simulink model "Q6_b"  (R2017a)
settings: Solver=FixedStepAuto  StartTime=0.0  StopTime=10  FixedStep=0.01  RelTol=0.00001
model workspace (MAT data in the model file):
  Kp_1 = 10000
  Kp_2 = 10000
  Kv_1 = 200
  Kv_2 = 200
  a_1 = 1
  a_2 = 1
  g = 9.8
  m_1 = 1
  m_2 = 1
  q1_0 = 0
  q1_dot_0 = 0
  q1_dot_f = 0
  q1_double_dot_0 = 0
  q1_double_dot_f = 0
  q1_f = 0.523598775598
  q2_0 = 0
  q2_dot_0 = 0
  q2_dot_f = 0
  q2_double_dot_0 = 0
  q2_double_dot_f = 0
  q2_f = 2.09439510239
  simulation_time = 4
libraries: simulink x25
settings Model: Creator=Omer  LastModifiedBy=Omer
settings ModelReferenceCC: ModelReferenceMinAlgLoopOccurrences=on

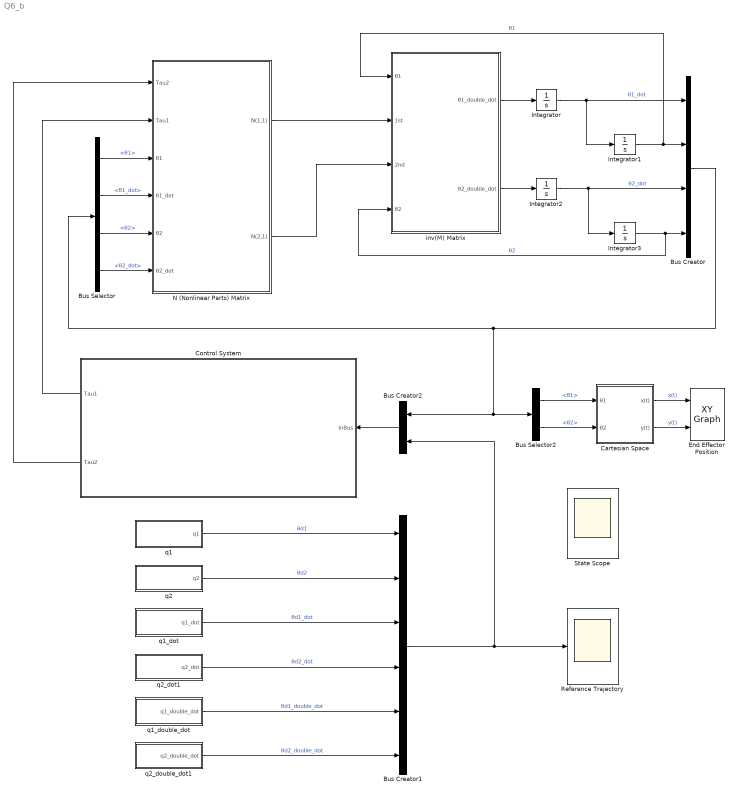
== system Q6_b ==
  Bus Creator : BusCreator  Inputs=4
  Bus Creator1 : BusCreator  Inputs=6
  Bus Creator2 : BusCreator  Inputs=2
  Bus Selector : BusSelector  OutputSignals=θ1,θ1_dot,θ2,θ2_dot
  Bus Selector2 : BusSelector  OutputSignals=θ1,θ2
  "Cartesian Space " : Subsystem  TreatAsAtomicUnit=on
  Control System : Subsystem  TreatAsAtomicUnit=on
  End Effector Position : simulink/Sinks/XY Graph  xmin=-1  xmax=3  ymin=-1  ymax=2  st=-1
  Integrator{,1..3} (4 alike) : Integrator
  N (Nonlinear Parts) Matrix : Subsystem  TreatAsAtomicUnit=on
  Reference Trajectory : Scope
  State Scope : Scope
      settings: Floating=on
  inv(M) Matrix : Subsystem  TreatAsAtomicUnit=on
  q1 : Subsystem  TreatAsAtomicUnit=on
  q1_dot : Subsystem  TreatAsAtomicUnit=on
  q1_double_dot : Subsystem  TreatAsAtomicUnit=on
  q2 : Subsystem  TreatAsAtomicUnit=on
  q2_dot1 : Subsystem  TreatAsAtomicUnit=on
  q2_double_dot1 : Subsystem  TreatAsAtomicUnit=on
  wires:
  N (Nonlinear Parts) Matrix/2(N(2,1)) -> inv(M) Matrix/3(2nd)
  N (Nonlinear Parts) Matrix/1(N(1,1)) -> inv(M) Matrix/2(1st)
  Bus Creator/1 -> Bus Selector/1, Bus Creator2/1, Bus Selector2/1
  inv(M) Matrix/2(θ2_double_dot) -> Integrator2/1
  Bus Selector/1 -> N (Nonlinear Parts) Matrix/3("θ1 ")  "<θ1>"
  Integrator2/1 -> Integrator3/1, Bus Creator/3  "θ2_dot"
  Integrator3/1 -> inv(M) Matrix/4(θ2), Bus Creator/4  "θ2"
  Integrator1/1 -> inv(M) Matrix/1(θ1), Bus Creator/2  "θ1"
  Bus Selector/3 -> N (Nonlinear Parts) Matrix/5(θ2)  "<θ2>"
  Bus Selector/2 -> N (Nonlinear Parts) Matrix/4(θ1_dot)  "<θ1_dot>"
  Integrator/1 -> Bus Creator/1, Integrator1/1  "θ1_dot"
  Bus Selector/4 -> N (Nonlinear Parts) Matrix/6(θ2_dot)  "<θ2_dot>"
  inv(M) Matrix/1(θ1_double_dot) -> Integrator/1
  Bus Selector2/1 -> "Cartesian Space "/1(θ1)  "<θ1>"
  Bus Selector2/2 -> "Cartesian Space "/2(θ2)  "<θ2>"
  "Cartesian Space "/1(x(t)) -> End Effector Position/1  "x(t)"
  "Cartesian Space "/2(y(t)) -> End Effector Position/2  "y(t)"
  Bus Creator2/1 -> Control System/1(InBus)
  Bus Creator1/1 -> Bus Creator2/2, Reference Trajectory/1
  q1/1(q1) -> Bus Creator1/1  "θd1"
  q2/1(q2) -> Bus Creator1/2  "θd2"
  Control System/2(Tau2) -> N (Nonlinear Parts) Matrix/1(Tau2)
  Control System/1(Tau1) -> N (Nonlinear Parts) Matrix/2(Tau1)
  q1_dot/1(q1_dot) -> Bus Creator1/3  "θd1_dot"
  q2_dot1/1(q2_dot) -> Bus Creator1/4  "θd2_dot"
  q1_double_dot/1(q1_double_dot) -> Bus Creator1/5  "θd1_double_dot"
  q2_double_dot1/1(q2_double_dot) -> Bus Creator1/6  "θd2_double_dot"

== system Q6_b/Cartesian Space  ==
  θ1 : Inport
  θ2 : Inport  Port=2
  Gain : Gain  Gain=a_1
  Gain1 : Gain  Gain=a_1
  Gain2 : Gain  Gain=a_2
  Gain3 : Gain  Gain=a_2
  Sum : Sum  Inputs=++|
  Sum1 : Sum  Inputs=|++
  Sum2 : Sum  Inputs=+|+
  Trig Func : Trigonometry
  Trig Func1 : Trigonometry
  Trig Func2 : Trigonometry  Operator=cos
  Trig Func3 : Trigonometry  Operator=cos
  x(t) : Outport
  y(t) : Outport  Port=2
  wires:
  θ1/1 -> Trig Func2/1, Trig Func/1, Sum/1
  θ2/1 -> Sum/2
  Sum/1 -> Trig Func3/1, Trig Func1/1
  Sum2/1 -> y(t)/1
  Sum1/1 -> x(t)/1
  Trig Func/1 -> Gain/1
  Gain/1 -> Sum2/1
  Trig Func2/1 -> Gain1/1
  Gain1/1 -> Sum1/1
  Trig Func1/1 -> Gain2/1
  Gain2/1 -> Sum2/2
  Trig Func3/1 -> Gain3/1
  Gain3/1 -> Sum1/2

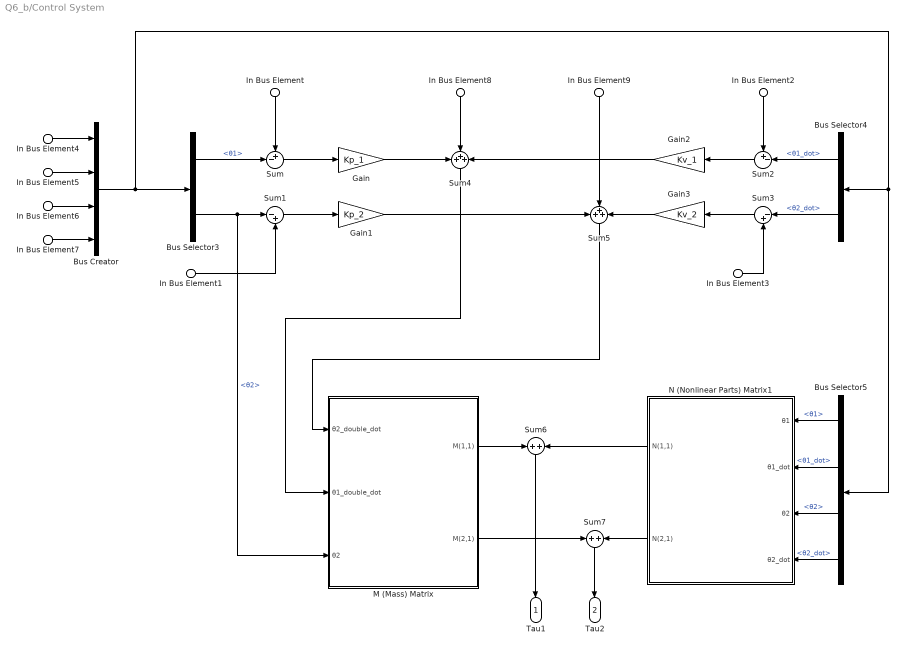
== system Q6_b/Control System ==
  In Bus Element : Inport  PortName=InBus  Element=signal2.θd1
  In Bus Element1 : Inport  PortName=InBus  Element=signal2.θd2
  In Bus Element2 : Inport  PortName=InBus  Element=signal2.θd1_dot
  In Bus Element3 : Inport  PortName=InBus  Element=signal2.θd2_dot
  In Bus Element8 : Inport  PortName=InBus  Element=signal2.θd1_double_dot
  In Bus Element9 : Inport  PortName=InBus  Element=signal2.θd2_double_dot
  In Bus Element4 : Inport  PortName=InBus  Element=signal1.θ1_dot
  In Bus Element5 : Inport  PortName=InBus  Element=signal1.θ1
  In Bus Element6 : Inport  PortName=InBus  Element=signal1.θ2_dot
  In Bus Element7 : Inport  PortName=InBus  Element=signal1.θ2
  Bus Creator : BusCreator  Inputs=4
  Bus Selector3 : BusSelector  OutputSignals=θ1,θ2
  Bus Selector4 : BusSelector  OutputSignals=θ1_dot,θ2_dot
  Bus Selector5 : BusSelector  OutputSignals=θ1,θ1_dot,θ2,θ2_dot
  Gain : Gain  Gain=Kp_1
  Gain1 : Gain  Gain=Kp_2
  Gain2 : Gain  Gain=Kv_1
  Gain3 : Gain  Gain=Kv_2
  M (Mass) Matrix : Subsystem  TreatAsAtomicUnit=on
  N (Nonlinear Parts) Matrix1 : Subsystem  TreatAsAtomicUnit=on
  Sum : Sum  Inputs=+-|
  Sum1 : Sum  Inputs=|-+
  Sum2 : Sum  Inputs=+-|
  Sum3 : Sum  Inputs=|-+
  Sum4 : Sum  Inputs=+++
  Sum5 : Sum  Inputs=+++
  Sum6 : Sum  Inputs=+|+
  Sum7 : Sum  Inputs=+|+
  Tau1 : Outport
  Tau2 : Outport  Port=2
  wires:
  Sum4/1 -> M (Mass) Matrix/2(θ1_double_dot)
  M (Mass) Matrix/1(M(1,1)) -> Sum6/1
  In Bus Element1/1 -> Sum1/2
  Sum7/1 -> Tau2/1
  In Bus Element7/1 -> Bus Creator/4
  In Bus Element3/1 -> Sum3/2
  N (Nonlinear Parts) Matrix1/1(N(1,1)) -> Sum6/2
  In Bus Element5/1 -> Bus Creator/2
  Gain1/1 -> Sum5/1
  In Bus Element4/1 -> Bus Creator/1
  Sum3/1 -> Gain3/1
  Sum2/1 -> Gain2/1
  In Bus Element2/1 -> Sum2/1
  Bus Selector5/2 -> N (Nonlinear Parts) Matrix1/2(θ1_dot)  "<θ1_dot>"
  Sum/1 -> Gain/1
  Bus Selector5/3 -> N (Nonlinear Parts) Matrix1/3(θ2)  "<θ2>"
  Sum5/1 -> M (Mass) Matrix/1(θ2_double_dot)
  M (Mass) Matrix/2(M(2,1)) -> Sum7/1
  Bus Selector5/4 -> N (Nonlinear Parts) Matrix1/4(θ2_dot)  "<θ2_dot>"
  Bus Selector4/1 -> Sum2/2  "<θ1_dot>"
  Sum6/1 -> Tau1/1
  Gain/1 -> Sum4/1
  In Bus Element8/1 -> Sum4/2
  In Bus Element9/1 -> Sum5/2
  Bus Selector5/1 -> N (Nonlinear Parts) Matrix1/1("θ1 ")  "<θ1>"
  Gain2/1 -> Sum4/3
  In Bus Element6/1 -> Bus Creator/3
  In Bus Element/1 -> Sum/1
  Gain3/1 -> Sum5/3
  Bus Selector3/2 -> M (Mass) Matrix/3(θ2), Sum1/1  "<θ2>"
  Bus Selector3/1 -> Sum/2  "<θ1>"
  N (Nonlinear Parts) Matrix1/2(N(2,1)) -> Sum7/2
  Bus Selector4/2 -> Sum3/1  "<θ2_dot>"
  Sum1/1 -> Gain1/1
  Bus Creator/1 -> Bus Selector3/1, Bus Selector4/1, Bus Selector5/1

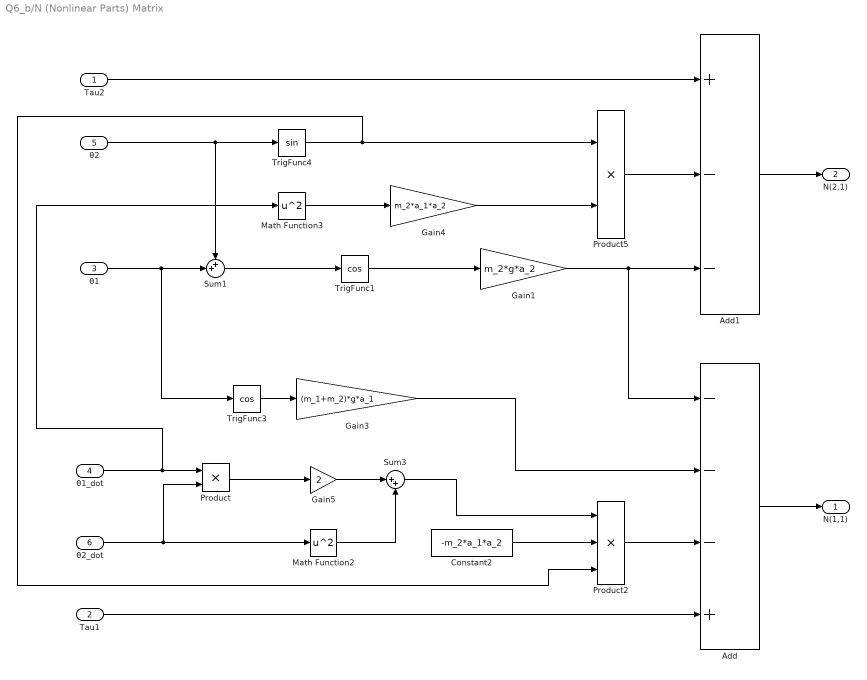
== system Q6_b/N (Nonlinear Parts) Matrix ==
  Tau2 : Inport
  Tau1 : Inport  Port=2
  "θ1 " : Inport  Port=3
  θ1_dot : Inport  Port=4
  θ2 : Inport  Port=5
  θ2_dot : Inport  Port=6
  Add : Sum  Inputs=---+
  Add1 : Sum  Inputs=+--
  Constant2 : Constant  Value=-m_2*a_1*a_2
  Gain1 : Gain  Gain=m_2*g*a_2
  Gain3 : Gain  Gain=(m_1+m_2)*g*a_1
  Gain4 : Gain  Gain=m_2*a_1*a_2
  Gain5 : Gain  Gain=2
  Math Function2 : Math  Operator=square  SaturateOnIntegerOverflow=on
  Math Function3 : Math  Operator=square  SaturateOnIntegerOverflow=on
  Product : Product
  Product2 : Product  Inputs=3
  Product5 : Product
  Sum1 : Sum  Inputs=++|
  Sum3 : Sum  Inputs=|++
  TrigFunc1 : Trigonometry  Operator=cos
  TrigFunc3 : Trigonometry  Operator=cos
  TrigFunc4 : Trigonometry
  N(1,1) : Outport
  N(2,1) : Outport  Port=2
  wires:
  Product2/1 -> Add/3
  Gain3/1 -> Add/2
  θ2/1 -> TrigFunc4/1, Sum1/1
  TrigFunc4/1 -> Product2/3, Product5/1
  Add1/1 -> N(2,1)/1
  Math Function3/1 -> Gain4/1
  θ1_dot/1 -> Product/1, Math Function3/1
  θ2_dot/1 -> Product/2, Math Function2/1
  Sum1/1 -> TrigFunc1/1
  Add/1 -> N(1,1)/1
  Sum3/1 -> Product2/1
  Math Function2/1 -> Sum3/2
  Tau2/1 -> Add1/1
  Constant2/1 -> Product2/2
  TrigFunc3/1 -> Gain3/1
  TrigFunc1/1 -> Gain1/1
  "θ1 "/1 -> TrigFunc3/1, Sum1/2
  Product5/1 -> Add1/2
  Tau1/1 -> Add/4
  Gain4/1 -> Product5/2
  Gain1/1 -> Add1/3, Add/1
  Product/1 -> Gain5/1
  Gain5/1 -> Sum3/1

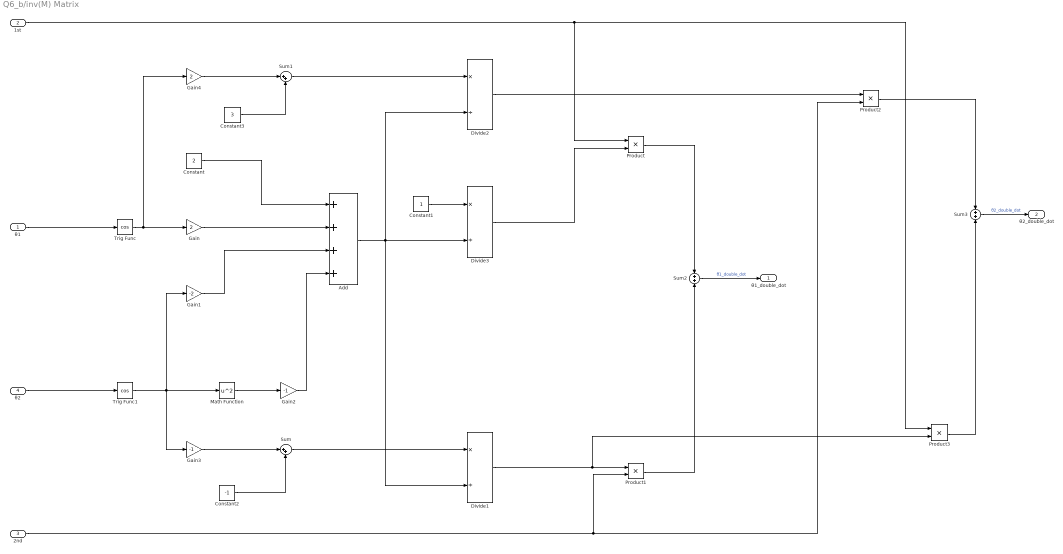
== system Q6_b/inv(M) Matrix ==
  θ1 : Inport
  1st : Inport  Port=2
  2nd : Inport  Port=3
  θ2 : Inport  Port=4
  Add : Sum  Inputs=4
  Constant : Constant  Value=2
  Constant1 : Constant
  Constant2 : Constant  Value=-1
  Constant3 : Constant  Value=3
  Divide1 : Product  Inputs=*/
  Divide2 : Product  Inputs=*/
  Divide3 : Product  Inputs=*/
  Gain : Gain  Gain=2
  Gain1 : Gain  Gain=-2
  Gain2 : Gain  Gain=-1
  Gain3 : Gain  Gain=-1
  Gain4 : Gain  Gain=2
  Math Function : Math  Operator=square  SaturateOnIntegerOverflow=on
  Product{,1..3} (4 alike) : Product
  Sum : Sum  Inputs=|++
  Sum1 : Sum  Inputs=|++
  Sum2 : Sum  Inputs=+|+
  Sum3 : Sum  Inputs=+|+
  Trig Func : Trigonometry  Operator=cos
  Trig Func1 : Trigonometry  Operator=cos
  θ1_double_dot : Outport
  θ2_double_dot : Outport  Port=2
  wires:
  Add/1 -> Divide2/2, Divide3/2, Divide1/2
  θ1/1 -> Trig Func/1
  θ2/1 -> Trig Func1/1
  Trig Func1/1 -> Gain3/1, Gain1/1, Math Function/1
  Trig Func/1 -> Gain4/1, Gain/1
  Constant/1 -> Add/1
  Gain/1 -> Add/2
  Gain1/1 -> Add/3
  Constant1/1 -> Divide3/1
  Math Function/1 -> Gain2/1
  Gain2/1 -> Add/4
  Gain3/1 -> Sum/1
  Constant2/1 -> Sum/2
  Sum/1 -> Divide1/1
  Constant3/1 -> Sum1/2
  Gain4/1 -> Sum1/1
  1st/1 -> Product/1, Product3/1
  Divide3/1 -> Product/2
  Divide1/1 -> Product3/2, Product1/1
  2nd/1 -> Product2/2, Product1/2
  Product/1 -> Sum2/1
  Product1/1 -> Sum2/2
  Sum2/1 -> θ1_double_dot/1  "θ1_double_dot"
  Sum1/1 -> Divide2/1
  Divide2/1 -> Product2/1
  Product2/1 -> Sum3/1
  Sum3/1 -> θ2_double_dot/1  "θ2_double_dot"
  Product3/1 -> Sum3/2

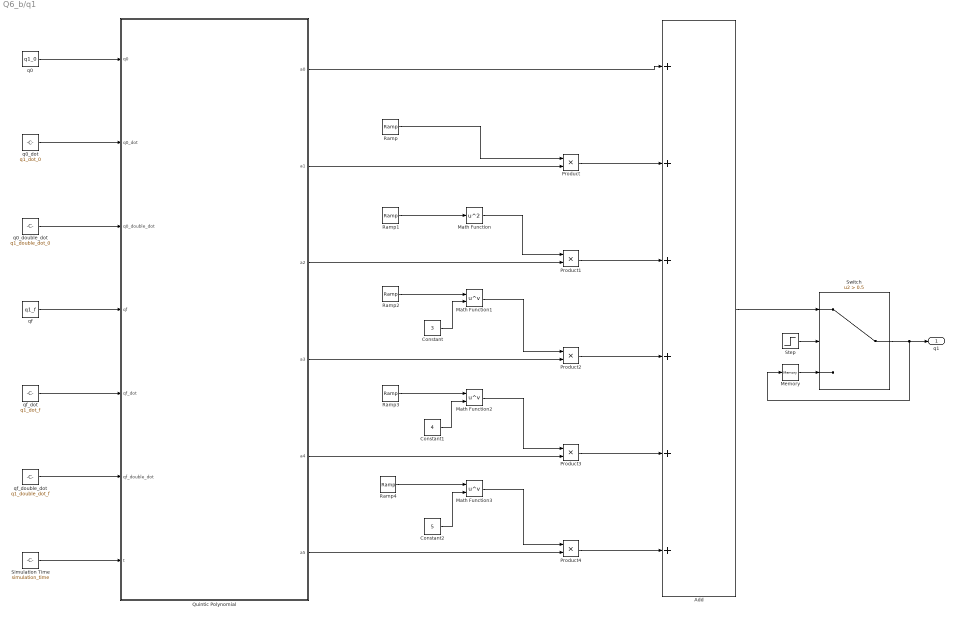
== system Q6_b/q1 ==
  Add : Sum  Inputs=6
  Constant : Constant  Value=3
  Constant1 : Constant  Value=4
  Constant2 : Constant  Value=5
  Math Function : Math  Operator=square  SaturateOnIntegerOverflow=on
  Math Function1 : Math  Operator=pow  SaturateOnIntegerOverflow=on
  Math Function2 : Math  Operator=pow  SaturateOnIntegerOverflow=on
  Math Function3 : Math  Operator=pow  SaturateOnIntegerOverflow=on
  Memory : Memory
  Product{,1..4} (5 alike) : Product
  Quintic Polynomial : MATLAB Function  TreatAsAtomicUnit=on
  Ramp{,1..4} (5 alike) : simulink/Sources/Ramp  slope=1  start=0  X0=0
  Simulation Time : Constant  Value=simulation_time
  Step : Step  Time=simulation_time  Before=1  After=0  SampleTime=0
  Switch : Switch  Criteria=u2 > Threshold  Threshold=0.5
  q0 : Constant  Value=q1_0
  q0_dot : Constant  Value=q1_dot_0
  q0_double_dot : Constant  Value=q1_double_dot_0
  qf : Constant  Value=q1_f
  qf_dot : Constant  Value=q1_dot_f
  qf_double_dot : Constant  Value=q1_double_dot_f
  q1 : Outport
  wires:
  Ramp1/1 -> Math Function/1
  Product4/1 -> Add/6
  Product/1 -> Add/2
  Product2/1 -> Add/4
  Math Function/1 -> Product1/1
  Quintic Polynomial/1(a0) -> Add/1
  Quintic Polynomial/2(a1) -> Product/2
  Product3/1 -> Add/5
  Simulation Time/1 -> Quintic Polynomial/7(t)
  Ramp/1 -> Product/1
  qf_dot/1 -> Quintic Polynomial/5(qf_dot)
  qf_double_dot/1 -> Quintic Polynomial/6(qf_double_dot)
  qf/1 -> Quintic Polynomial/4(qf)
  Ramp3/1 -> Math Function2/1
  Math Function2/1 -> Product3/1
  q0_double_dot/1 -> Quintic Polynomial/3(q0_double_dot)
  Constant2/1 -> Math Function3/2
  Quintic Polynomial/4(a3) -> Product2/2
  q0_dot/1 -> Quintic Polynomial/2(q0_dot)
  Ramp4/1 -> Math Function3/1
  Quintic Polynomial/5(a4) -> Product3/2
  Constant1/1 -> Math Function2/2
  Quintic Polynomial/6(a5) -> Product4/2
  Product1/1 -> Add/3
  Constant/1 -> Math Function1/2
  q0/1 -> Quintic Polynomial/1(q0)
  Math Function3/1 -> Product4/1
  Quintic Polynomial/3(a2) -> Product1/2
  Ramp2/1 -> Math Function1/1
  Math Function1/1 -> Product2/1
  Memory/1 -> Switch/3
  Switch/1 -> Memory/1, q1/1
  Add/1 -> Switch/1
  Step/1 -> Switch/2

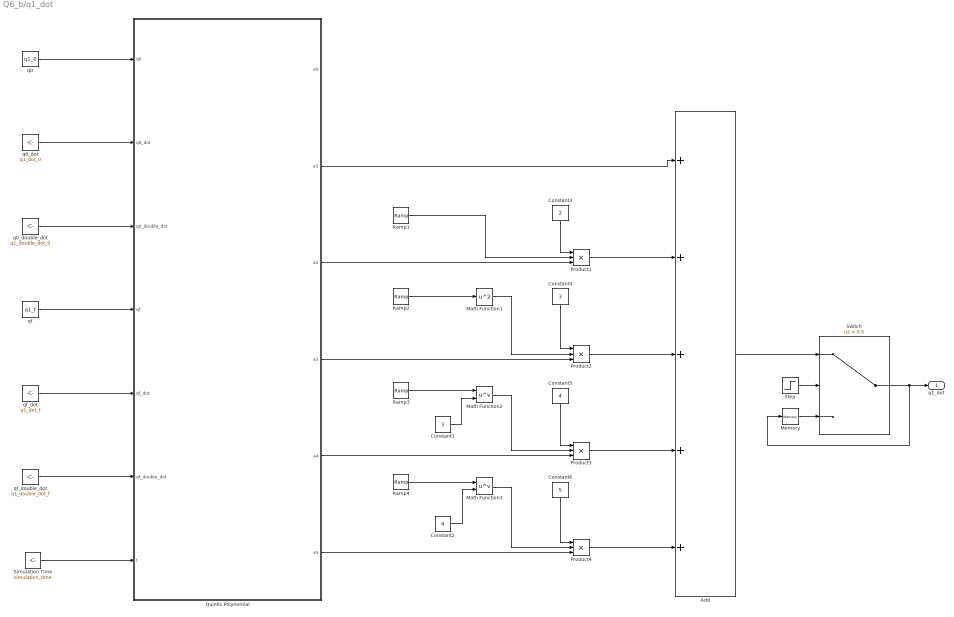
== system Q6_b/q1_dot ==
  Add : Sum  Inputs=5
  Constant1 : Constant  Value=3
  Constant2 : Constant  Value=4
  Constant3 : Constant  Value=2
  Constant4 : Constant  Value=3
  Constant5 : Constant  Value=4
  Constant6 : Constant  Value=5
  Math Function1 : Math  Operator=square  SaturateOnIntegerOverflow=on
  Math Function2 : Math  Operator=pow  SaturateOnIntegerOverflow=on
  Math Function3 : Math  Operator=pow  SaturateOnIntegerOverflow=on
  Memory : Memory
  Product{1..4} (4 alike) : Product  Inputs=3
  Quintic Polynomial : MATLAB Function  TreatAsAtomicUnit=on
  Ramp{1..4} (4 alike) : simulink/Sources/Ramp  slope=1  start=0  X0=0
  Simulation Time : Constant  Value=simulation_time
  Step : Step  Time=simulation_time  Before=1  After=0  SampleTime=0
  Switch : Switch  Criteria=u2 > Threshold  Threshold=0.5
  q0 : Constant  Value=q1_0
  q0_dot : Constant  Value=q1_dot_0
  q0_double_dot : Constant  Value=q1_double_dot_0
  qf : Constant  Value=q1_f
  qf_dot : Constant  Value=q1_dot_f
  qf_double_dot : Constant  Value=q1_double_dot_f
  q1_dot : Outport
  wires:
  Constant6/1 -> Product4/1
  Ramp1/1 -> Product1/2
  Ramp3/1 -> Math Function2/1
  Product1/1 -> Add/2
  Math Function1/1 -> Product2/2
  Simulation Time/1 -> Quintic Polynomial/7(t)
  Ramp4/1 -> Math Function3/1
  qf_double_dot/1 -> Quintic Polynomial/6(qf_double_dot)
  Quintic Polynomial/6(a5) -> Product4/3
  q0_double_dot/1 -> Quintic Polynomial/3(q0_double_dot)
  Product2/1 -> Add/3
  Quintic Polynomial/4(a3) -> Product2/3
  q0_dot/1 -> Quintic Polynomial/2(q0_dot)
  q0/1 -> Quintic Polynomial/1(q0)
  Quintic Polynomial/2(a1) -> Add/1
  Ramp2/1 -> Math Function1/1
  Math Function2/1 -> Product3/2
  Constant5/1 -> Product3/1
  Constant4/1 -> Product2/1
  Product3/1 -> Add/4
  Math Function3/1 -> Product4/2
  qf_dot/1 -> Quintic Polynomial/5(qf_dot)
  Constant3/1 -> Product1/1
  Constant1/1 -> Math Function2/2
  Constant2/1 -> Math Function3/2
  Product4/1 -> Add/5
  Quintic Polynomial/5(a4) -> Product3/3
  qf/1 -> Quintic Polynomial/4(qf)
  Quintic Polynomial/3(a2) -> Product1/3
  Memory/1 -> Switch/3
  Add/1 -> Switch/1
  Switch/1 -> q1_dot/1, Memory/1
  Step/1 -> Switch/2

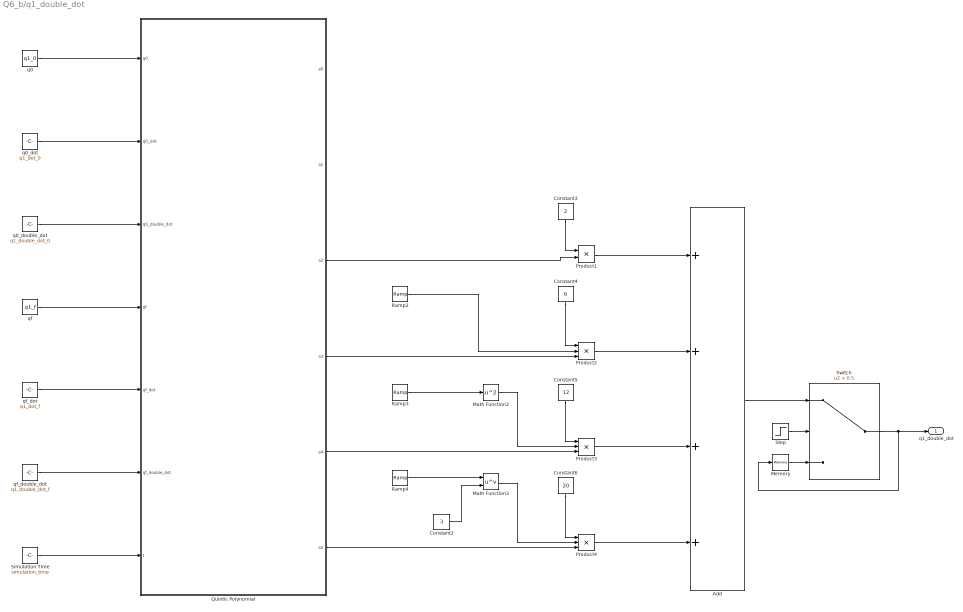
== system Q6_b/q1_double_dot ==
  Add : Sum  Inputs=4
  Constant2 : Constant  Value=3
  Constant3 : Constant  Value=2
  Constant4 : Constant  Value=6
  Constant5 : Constant  Value=12
  Constant6 : Constant  Value=20
  Math Function2 : Math  Operator=square  SaturateOnIntegerOverflow=on
  Math Function3 : Math  Operator=pow  SaturateOnIntegerOverflow=on
  Memory : Memory
  Product1 : Product
  Product2 : Product  Inputs=3
  Product3 : Product  Inputs=3
  Product4 : Product  Inputs=3
  Quintic Polynomial : MATLAB Function  TreatAsAtomicUnit=on
  Ramp2 : simulink/Sources/Ramp  slope=1  start=0  X0=0
  Ramp3 : simulink/Sources/Ramp  slope=1  start=0  X0=0
  Ramp4 : simulink/Sources/Ramp  slope=1  start=0  X0=0
  Simulation Time : Constant  Value=simulation_time
  Step : Step  Time=simulation_time  Before=1  After=0  SampleTime=0
  Switch : Switch  Criteria=u2 > Threshold  Threshold=0.5
  q0 : Constant  Value=q1_0
  q0_dot : Constant  Value=q1_dot_0
  q0_double_dot : Constant  Value=q1_double_dot_0
  qf : Constant  Value=q1_f
  qf_dot : Constant  Value=q1_dot_f
  qf_double_dot : Constant  Value=q1_double_dot_f
  q1_double_dot : Outport
  wires:
  Quintic Polynomial/6(a5) -> Product4/3
  Quintic Polynomial/5(a4) -> Product3/3
  Quintic Polynomial/4(a3) -> Product2/3
  Quintic Polynomial/3(a2) -> Product1/2
  q0_dot/1 -> Quintic Polynomial/2(q0_dot)
  Constant4/1 -> Product2/1
  Constant5/1 -> Product3/1
  Constant6/1 -> Product4/1
  Math Function3/1 -> Product4/2
  Product1/1 -> Add/1
  Constant3/1 -> Product1/1
  Math Function2/1 -> Product3/2
  Product2/1 -> Add/2
  Ramp2/1 -> Product2/2
  Ramp4/1 -> Math Function3/1
  Product3/1 -> Add/3
  qf/1 -> Quintic Polynomial/4(qf)
  qf_dot/1 -> Quintic Polynomial/5(qf_dot)
  Product4/1 -> Add/4
  q0/1 -> Quintic Polynomial/1(q0)
  Constant2/1 -> Math Function3/2
  q0_double_dot/1 -> Quintic Polynomial/3(q0_double_dot)
  Ramp3/1 -> Math Function2/1
  qf_double_dot/1 -> Quintic Polynomial/6(qf_double_dot)
  Simulation Time/1 -> Quintic Polynomial/7(t)
  Memory/1 -> Switch/3
  Add/1 -> Switch/1
  Switch/1 -> q1_double_dot/1, Memory/1
  Step/1 -> Switch/2

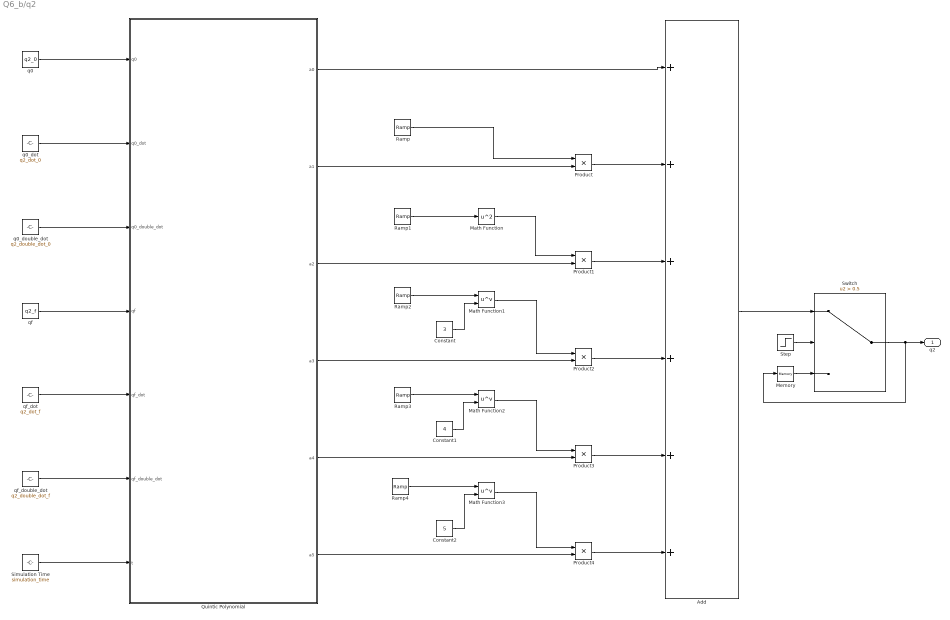
== system Q6_b/q2 ==
  Add : Sum  Inputs=6
  Constant : Constant  Value=3
  Constant1 : Constant  Value=4
  Constant2 : Constant  Value=5
  Math Function : Math  Operator=square  SaturateOnIntegerOverflow=on
  Math Function1 : Math  Operator=pow  SaturateOnIntegerOverflow=on
  Math Function2 : Math  Operator=pow  SaturateOnIntegerOverflow=on
  Math Function3 : Math  Operator=pow  SaturateOnIntegerOverflow=on
  Memory : Memory
  Product{,1..4} (5 alike) : Product
  Quintic Polynomial : MATLAB Function  TreatAsAtomicUnit=on
  Ramp{,1..4} (5 alike) : simulink/Sources/Ramp  slope=1  start=0  X0=0
  Simulation Time : Constant  Value=simulation_time
  Step : Step  Time=simulation_time  Before=1  After=0  SampleTime=0
  Switch : Switch  Criteria=u2 > Threshold  Threshold=0.5
  q0 : Constant  Value=q2_0
  q0_dot : Constant  Value=q2_dot_0
  q0_double_dot : Constant  Value=q2_double_dot_0
  qf : Constant  Value=q2_f
  qf_dot : Constant  Value=q2_dot_f
  qf_double_dot : Constant  Value=q2_double_dot_f
  q2 : Outport
  wires:
  Ramp/1 -> Product/1
  Quintic Polynomial/2(a1) -> Product/2
  Quintic Polynomial/1(a0) -> Add/1
  Product/1 -> Add/2
  Product1/1 -> Add/3
  Product2/1 -> Add/4
  Product3/1 -> Add/5
  Product4/1 -> Add/6
  Ramp1/1 -> Math Function/1
  Math Function/1 -> Product1/1
  Ramp2/1 -> Math Function1/1
  Ramp3/1 -> Math Function2/1
  Ramp4/1 -> Math Function3/1
  Quintic Polynomial/3(a2) -> Product1/2
  Math Function1/1 -> Product2/1
  Math Function2/1 -> Product3/1
  Math Function3/1 -> Product4/1
  Quintic Polynomial/4(a3) -> Product2/2
  Quintic Polynomial/5(a4) -> Product3/2
  Quintic Polynomial/6(a5) -> Product4/2
  Constant/1 -> Math Function1/2
  Constant1/1 -> Math Function2/2
  Constant2/1 -> Math Function3/2
  q0/1 -> Quintic Polynomial/1(q0)
  q0_dot/1 -> Quintic Polynomial/2(q0_dot)
  q0_double_dot/1 -> Quintic Polynomial/3(q0_double_dot)
  qf/1 -> Quintic Polynomial/4(qf)
  qf_dot/1 -> Quintic Polynomial/5(qf_dot)
  qf_double_dot/1 -> Quintic Polynomial/6(qf_double_dot)
  Simulation Time/1 -> Quintic Polynomial/7(t)
  Memory/1 -> Switch/3
  Add/1 -> Switch/1
  Switch/1 -> q2/1, Memory/1
  Step/1 -> Switch/2

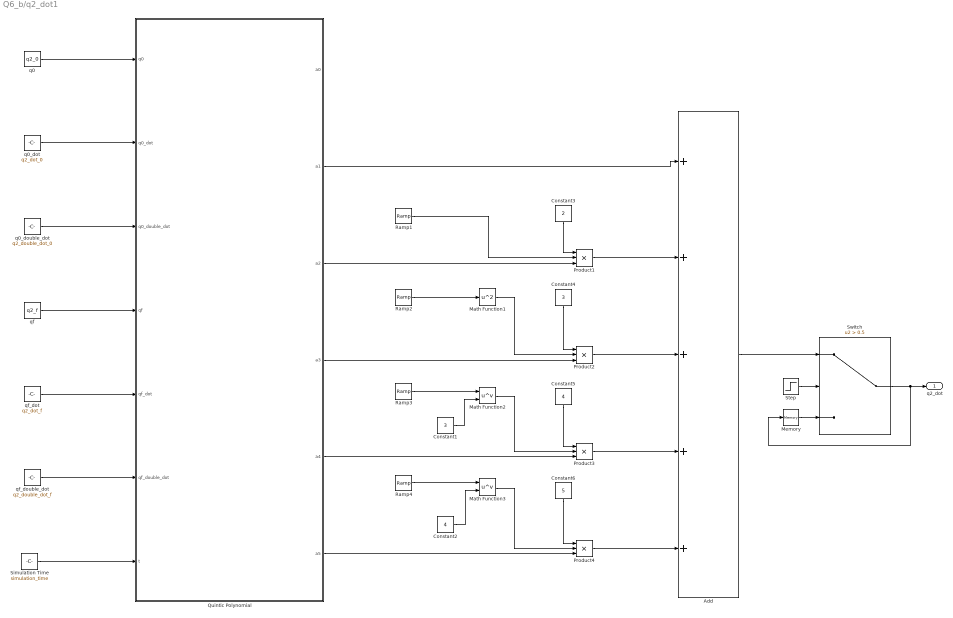
== system Q6_b/q2_dot1 ==
  Add : Sum  Inputs=5
  Constant1 : Constant  Value=3
  Constant2 : Constant  Value=4
  Constant3 : Constant  Value=2
  Constant4 : Constant  Value=3
  Constant5 : Constant  Value=4
  Constant6 : Constant  Value=5
  Math Function1 : Math  Operator=square  SaturateOnIntegerOverflow=on
  Math Function2 : Math  Operator=pow  SaturateOnIntegerOverflow=on
  Math Function3 : Math  Operator=pow  SaturateOnIntegerOverflow=on
  Memory : Memory
  Product{1..4} (4 alike) : Product  Inputs=3
  Quintic Polynomial : MATLAB Function  TreatAsAtomicUnit=on
  Ramp{1..4} (4 alike) : simulink/Sources/Ramp  slope=1  start=0  X0=0
  Simulation Time : Constant  Value=simulation_time
  Step : Step  Time=simulation_time  Before=1  After=0  SampleTime=0
  Switch : Switch  Criteria=u2 > Threshold  Threshold=0.5
  q0 : Constant  Value=q2_0
  q0_dot : Constant  Value=q2_dot_0
  q0_double_dot : Constant  Value=q2_double_dot_0
  qf : Constant  Value=q2_f
  qf_dot : Constant  Value=q2_dot_f
  qf_double_dot : Constant  Value=q2_double_dot_f
  q2_dot : Outport
  wires:
  Quintic Polynomial/2(a1) -> Add/1
  Product1/1 -> Add/2
  Product2/1 -> Add/3
  Product3/1 -> Add/4
  Product4/1 -> Add/5
  Ramp1/1 -> Product1/2
  Ramp2/1 -> Math Function1/1
  Ramp3/1 -> Math Function2/1
  Ramp4/1 -> Math Function3/1
  Quintic Polynomial/3(a2) -> Product1/3
  Math Function1/1 -> Product2/2
  Math Function2/1 -> Product3/2
  Math Function3/1 -> Product4/2
  Quintic Polynomial/4(a3) -> Product2/3
  Quintic Polynomial/5(a4) -> Product3/3
  Quintic Polynomial/6(a5) -> Product4/3
  Constant1/1 -> Math Function2/2
  Constant2/1 -> Math Function3/2
  q0/1 -> Quintic Polynomial/1(q0)
  q0_dot/1 -> Quintic Polynomial/2(q0_dot)
  q0_double_dot/1 -> Quintic Polynomial/3(q0_double_dot)
  qf/1 -> Quintic Polynomial/4(qf)
  qf_dot/1 -> Quintic Polynomial/5(qf_dot)
  qf_double_dot/1 -> Quintic Polynomial/6(qf_double_dot)
  Simulation Time/1 -> Quintic Polynomial/7(t)
  Constant3/1 -> Product1/1
  Constant4/1 -> Product2/1
  Constant5/1 -> Product3/1
  Constant6/1 -> Product4/1
  Memory/1 -> Switch/3
  Add/1 -> Switch/1
  Switch/1 -> q2_dot/1, Memory/1
  Step/1 -> Switch/2

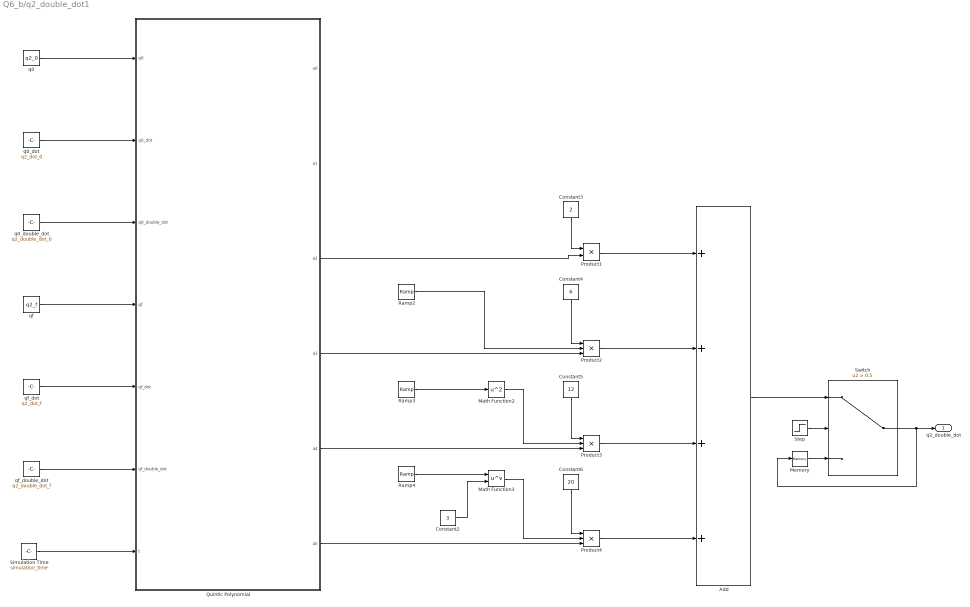
== system Q6_b/q2_double_dot1 ==
  Add : Sum  Inputs=4
  Constant2 : Constant  Value=3
  Constant3 : Constant  Value=2
  Constant4 : Constant  Value=6
  Constant5 : Constant  Value=12
  Constant6 : Constant  Value=20
  Math Function2 : Math  Operator=square  SaturateOnIntegerOverflow=on
  Math Function3 : Math  Operator=pow  SaturateOnIntegerOverflow=on
  Memory : Memory
  Product1 : Product
  Product2 : Product  Inputs=3
  Product3 : Product  Inputs=3
  Product4 : Product  Inputs=3
  Quintic Polynomial : MATLAB Function  TreatAsAtomicUnit=on
  Ramp2 : simulink/Sources/Ramp  slope=1  start=0  X0=0
  Ramp3 : simulink/Sources/Ramp  slope=1  start=0  X0=0
  Ramp4 : simulink/Sources/Ramp  slope=1  start=0  X0=0
  Simulation Time : Constant  Value=simulation_time
  Step : Step  Time=simulation_time  Before=1  After=0  SampleTime=0
  Switch : Switch  Criteria=u2 > Threshold  Threshold=0.5
  q0 : Constant  Value=q2_0
  q0_dot : Constant  Value=q2_dot_0
  q0_double_dot : Constant  Value=q2_double_dot_0
  qf : Constant  Value=q2_f
  qf_dot : Constant  Value=q2_dot_f
  qf_double_dot : Constant  Value=q2_double_dot_f
  q2_double_dot : Outport
  wires:
  Product1/1 -> Add/1
  Product2/1 -> Add/2
  Product3/1 -> Add/3
  Product4/1 -> Add/4
  Ramp3/1 -> Math Function2/1
  Ramp4/1 -> Math Function3/1
  Quintic Polynomial/3(a2) -> Product1/2
  Ramp2/1 -> Product2/2
  Math Function2/1 -> Product3/2
  Math Function3/1 -> Product4/2
  Quintic Polynomial/4(a3) -> Product2/3
  Quintic Polynomial/5(a4) -> Product3/3
  Quintic Polynomial/6(a5) -> Product4/3
  Constant2/1 -> Math Function3/2
  q0/1 -> Quintic Polynomial/1(q0)
  q0_dot/1 -> Quintic Polynomial/2(q0_dot)
  q0_double_dot/1 -> Quintic Polynomial/3(q0_double_dot)
  qf/1 -> Quintic Polynomial/4(qf)
  qf_dot/1 -> Quintic Polynomial/5(qf_dot)
  qf_double_dot/1 -> Quintic Polynomial/6(qf_double_dot)
  Simulation Time/1 -> Quintic Polynomial/7(t)
  Constant3/1 -> Product1/1
  Constant4/1 -> Product2/1
  Constant5/1 -> Product3/1
  Constant6/1 -> Product4/1
  Memory/1 -> Switch/3
  Add/1 -> Switch/1
  Switch/1 -> q2_double_dot/1, Memory/1
  Step/1 -> Switch/2

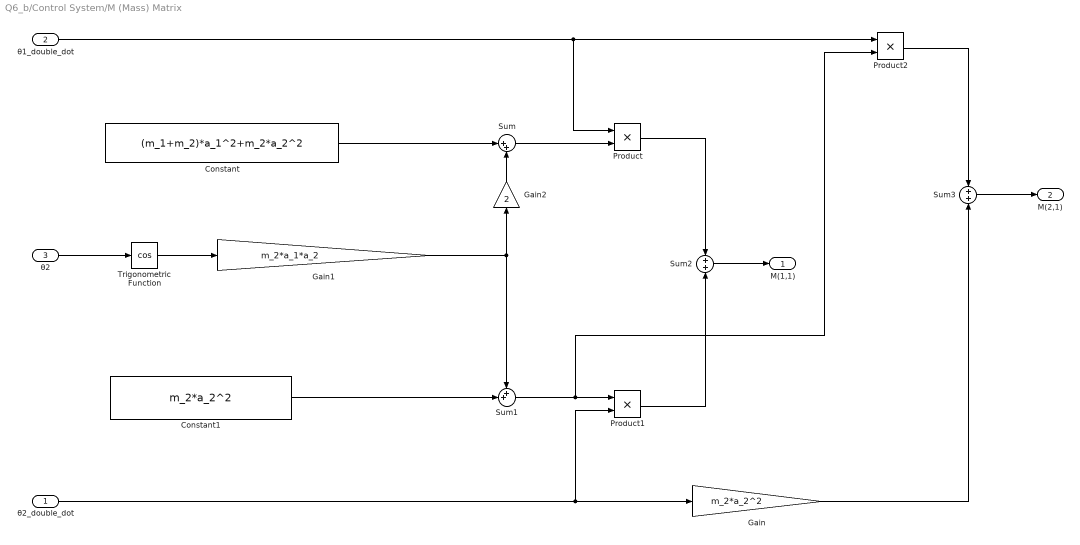
== system Q6_b/Control System/M (Mass) Matrix ==
  θ2_double_dot : Inport
  θ1_double_dot : Inport  Port=2
  θ2 : Inport  Port=3
  Constant : Constant  Value=(m_1+m_2)*a_1^2+m_2*a_2^2
  Constant1 : Constant  Value=m_2*a_2^2
  Gain : Gain  Gain=m_2*a_2^2
  Gain1 : Gain  Gain=m_2*a_1*a_2
  Gain2 : Gain  Gain=2
  Product : Product
  Product1 : Product
  Product2 : Product
  Sum : Sum  Inputs=|++
  Sum1 : Sum  Inputs=++|
  Sum2 : Sum  Inputs=+|+
  Sum3 : Sum  Inputs=+|+
  Trigonometric Function : Trigonometry  Operator=cos
  M(1,1) : Outport
  M(2,1) : Outport  Port=2
  wires:
  θ2/1 -> Trigonometric Function/1
  Trigonometric Function/1 -> Gain1/1
  Gain1/1 -> Gain2/1, Sum1/1
  Constant1/1 -> Sum1/2
  Constant/1 -> Sum/1
  θ1_double_dot/1 -> Product/1, Product2/1
  Sum/1 -> Product/2
  Sum1/1 -> Product2/2, Product1/1
  θ2_double_dot/1 -> Gain/1, Product1/2
  Product/1 -> Sum2/1
  Product1/1 -> Sum2/2
  Sum2/1 -> M(1,1)/1
  Product2/1 -> Sum3/1
  Gain/1 -> Sum3/2
  Sum3/1 -> M(2,1)/1
  Gain2/1 -> Sum/2

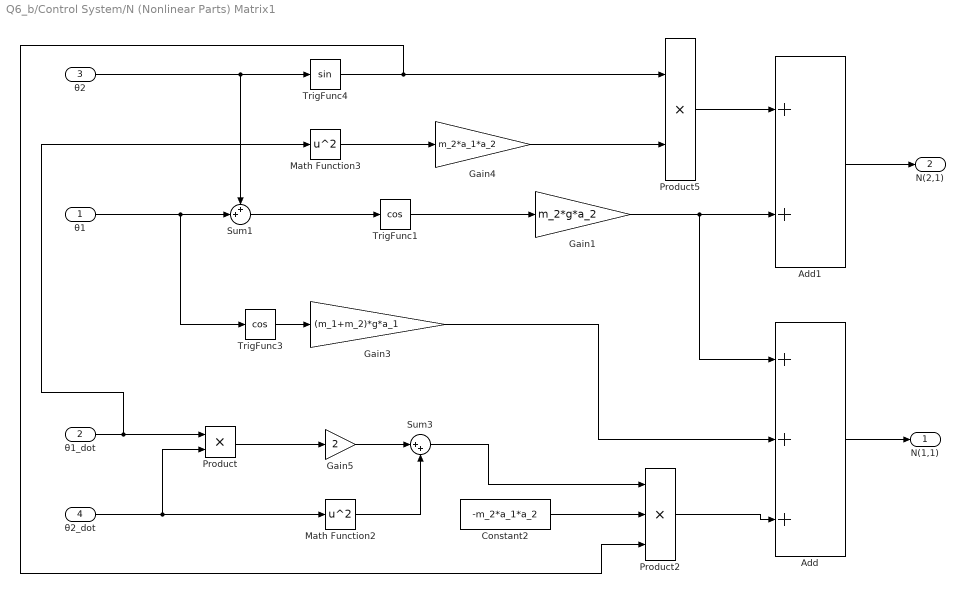
== system Q6_b/Control System/N (Nonlinear Parts) Matrix1 ==
  "θ1 " : Inport
  θ1_dot : Inport  Port=2
  θ2 : Inport  Port=3
  θ2_dot : Inport  Port=4
  Add : Sum  Inputs=+++
  Add1 : Sum
  Constant2 : Constant  Value=-m_2*a_1*a_2
  Gain1 : Gain  Gain=m_2*g*a_2
  Gain3 : Gain  Gain=(m_1+m_2)*g*a_1
  Gain4 : Gain  Gain=m_2*a_1*a_2
  Gain5 : Gain  Gain=2
  Math Function2 : Math  Operator=square  SaturateOnIntegerOverflow=on
  Math Function3 : Math  Operator=square  SaturateOnIntegerOverflow=on
  Product : Product
  Product2 : Product  Inputs=3
  Product5 : Product
  Sum1 : Sum  Inputs=++|
  Sum3 : Sum  Inputs=|++
  TrigFunc1 : Trigonometry  Operator=cos
  TrigFunc3 : Trigonometry  Operator=cos
  TrigFunc4 : Trigonometry
  N(1,1) : Outport
  N(2,1) : Outport  Port=2
  wires:
  Product2/1 -> Add/3
  Gain3/1 -> Add/2
  θ2/1 -> TrigFunc4/1, Sum1/1
  TrigFunc4/1 -> Product2/3, Product5/1
  Add1/1 -> N(2,1)/1
  Math Function3/1 -> Gain4/1
  θ1_dot/1 -> Product/1, Math Function3/1
  θ2_dot/1 -> Product/2, Math Function2/1
  Sum1/1 -> TrigFunc1/1
  Add/1 -> N(1,1)/1
  Sum3/1 -> Product2/1
  Math Function2/1 -> Sum3/2
  Constant2/1 -> Product2/2
  TrigFunc3/1 -> Gain3/1
  TrigFunc1/1 -> Gain1/1
  "θ1 "/1 -> TrigFunc3/1, Sum1/2
  Gain4/1 -> Product5/2
  Gain1/1 -> Add/1, Add1/2
  Product/1 -> Gain5/1
  Gain5/1 -> Sum3/1
  Product5/1 -> Add1/1

== matlab function Q6_b/q1/Quintic Polynomial ==
  data: q0 input; a0 output; a1 output; a2 output; a3 output; a4 output; a5 output; q0_dot input; q0_double_dot input; qf input; qf_dot input; qf_double_dot input; t input
function [a0, a1, a2, a3, a4, a5] = fcn(q0, q0_dot, q0_double_dot, qf, qf_dot, qf_double_dot, t)

T = [1 0 0 0 0 0;
     0 1 0 0 0 0;
     0 0 2 0 0 0;
     1 t t^2 t^3 t^4 t^5;
     0 1 2*t 3*t^2 4*t^3 5*t^4;
     0 0 2 6*t 12*t^2 20*t^3];

q = [q0, q0_dot, q0_double_dot, qf, qf_dot, qf_double_dot]';
Q = inv(T)*q;
a0=Q(1); a1=Q(2); a2=Q(3); a3=Q(4); a4=Q(5); a5=Q(6);

== matlab function Q6_b/q2/Quintic Polynomial ==
  data: q0 input; a0 output; a1 output; a2 output; a3 output; a4 output; a5 output; q0_dot input; q0_double_dot input; qf input; qf_dot input; qf_double_dot input; t input
function [a0, a1, a2, a3, a4, a5] = fcn(q0, q0_dot, q0_double_dot, qf, qf_dot, qf_double_dot, t)

T = [1 0 0 0 0 0;
     0 1 0 0 0 0;
     0 0 2 0 0 0;
     1 t t^2 t^3 t^4 t^5;
     0 1 2*t 3*t^2 4*t^3 5*t^4;
     0 0 2 6*t 12*t^2 20*t^3];

q = [q0, q0_dot, q0_double_dot, qf, qf_dot, qf_double_dot]';
Q = inv(T)*q;
a0=Q(1); a1=Q(2); a2=Q(3); a3=Q(4); a4=Q(5); a5=Q(6);

== matlab function Q6_b/q1_dot/Quintic Polynomial ==
  data: q0 input; a0 output; a1 output; a2 output; a3 output; a4 output; a5 output; q0_dot input; q0_double_dot input; qf input; qf_dot input; qf_double_dot input; t input
function [a0, a1, a2, a3, a4, a5] = fcn(q0, q0_dot, q0_double_dot, qf, qf_dot, qf_double_dot, t)

T = [1 0 0 0 0 0;
     0 1 0 0 0 0;
     0 0 2 0 0 0;
     1 t t^2 t^3 t^4 t^5;
     0 1 2*t 3*t^2 4*t^3 5*t^4;
     0 0 2 6*t 12*t^2 20*t^3];

q = [q0, q0_dot, q0_double_dot, qf, qf_dot, qf_double_dot]';
Q = inv(T)*q;
a0=Q(1); a1=Q(2); a2=Q(3); a3=Q(4); a4=Q(5); a5=Q(6);

== matlab function Q6_b/q2_dot1/Quintic Polynomial ==
  data: q0 input; a0 output; a1 output; a2 output; a3 output; a4 output; a5 output; q0_dot input; q0_double_dot input; qf input; qf_dot input; qf_double_dot input; t input
function [a0, a1, a2, a3, a4, a5] = fcn(q0, q0_dot, q0_double_dot, qf, qf_dot, qf_double_dot, t)

T = [1 0 0 0 0 0;
     0 1 0 0 0 0;
     0 0 2 0 0 0;
     1 t t^2 t^3 t^4 t^5;
     0 1 2*t 3*t^2 4*t^3 5*t^4;
     0 0 2 6*t 12*t^2 20*t^3];

q = [q0, q0_dot, q0_double_dot, qf, qf_dot, qf_double_dot]';
Q = inv(T)*q;
a0=Q(1); a1=Q(2); a2=Q(3); a3=Q(4); a4=Q(5); a5=Q(6);

== matlab function Q6_b/q1_double_dot/Quintic Polynomial ==
  data: q0 input; a0 output; a1 output; a2 output; a3 output; a4 output; a5 output; q0_dot input; q0_double_dot input; qf input; qf_dot input; qf_double_dot input; t input
function [a0, a1, a2, a3, a4, a5] = fcn(q0, q0_dot, q0_double_dot, qf, qf_dot, qf_double_dot, t)

T = [1 0 0 0 0 0;
     0 1 0 0 0 0;
     0 0 2 0 0 0;
     1 t t^2 t^3 t^4 t^5;
     0 1 2*t 3*t^2 4*t^3 5*t^4;
     0 0 2 6*t 12*t^2 20*t^3];

q = [q0, q0_dot, q0_double_dot, qf, qf_dot, qf_double_dot]';
Q = inv(T)*q;
a0=Q(1); a1=Q(2); a2=Q(3); a3=Q(4); a4=Q(5); a5=Q(6);

== matlab function Q6_b/q2_double_dot1/Quintic Polynomial ==
  data: q0 input; a0 output; a1 output; a2 output; a3 output; a4 output; a5 output; q0_dot input; q0_double_dot input; qf input; qf_dot input; qf_double_dot input; t input
function [a0, a1, a2, a3, a4, a5] = fcn(q0, q0_dot, q0_double_dot, qf, qf_dot, qf_double_dot, t)

T = [1 0 0 0 0 0;
     0 1 0 0 0 0;
     0 0 2 0 0 0;
     1 t t^2 t^3 t^4 t^5;
     0 1 2*t 3*t^2 4*t^3 5*t^4;
     0 0 2 6*t 12*t^2 20*t^3];

q = [q0, q0_dot, q0_double_dot, qf, qf_dot, qf_double_dot]';
Q = inv(T)*q;
a0=Q(1); a1=Q(2); a2=Q(3); a3=Q(4); a4=Q(5); a5=Q(6);
